simulink subsystem "Find_Point_Coefficients"  (R2023b)
settings: Solver=VariableStepAuto  StartTime=0.0  StopTime=10.0  RelTol=1e-3
settings Model: Creator=FIRSTMentor  LastModifiedBy=FIRSTMentor

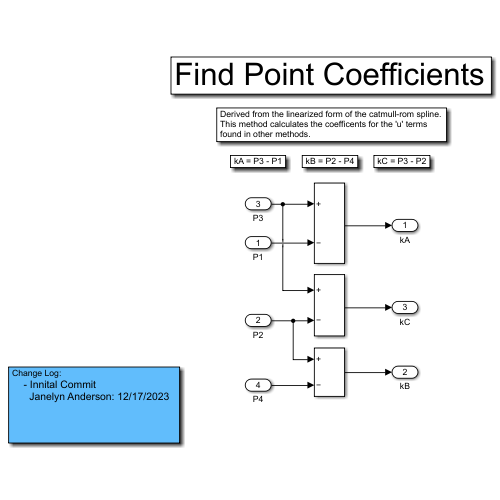
[thumbnail: Simulink's stored preview of the top-level diagram]
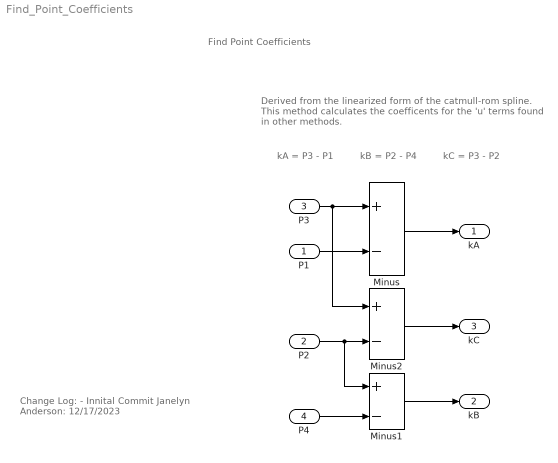
== system Find_Point_Coefficients ==
  note: kA = P3 - P1
  note: Derived from the linearized form of the catmull-rom spline. This method calculates the coefficents for the 'u' terms found in other methods.
  note: Find Point Coefficients
  note: Change Log:
      | - Innital Commit
      | Janelyn Anderson: 12/17/2023
  note: kB = P2 - P4
  note: kC = P3 - P2
  P1 : Inport
  P2 : Inport  Port=2
  P3 : Inport  Port=3
  P4 : Inport  Port=4
  Minus : Sum  Inputs=+-
  Minus1 : Sum  Inputs=+-
  Minus2 : Sum  Inputs=+-
  kA : Outport
  kB : Outport  Port=2
  kC : Outport  Port=3
  wires:
  P1/1 -> Minus/2
  P2/1 -> Minus2/2, Minus1/1
  Minus2/1 -> kC/1
  P4/1 -> Minus1/2
  P3/1 -> Minus2/1, Minus/1
  Minus1/1 -> kB/1
  Minus/1 -> kA/1
